simulink model "priority_01_prove"  (R2014b)
settings: Solver=FixedStepDiscrete  StartTime=0.0  StopTime=10.0  FixedStep=0.01  RelTol=1e-3
undefined symbols (not defined in the file): sldvsubsys
libraries: sldvlib x20, simulink x4
settings Model: Creator=Natasha  LastModifiedBy=JYOGANAN
settings DebuggingCC: UnderspecifiedInitializationDetection=Classic  MergeDetectMultiDrivingBlocksExec=none

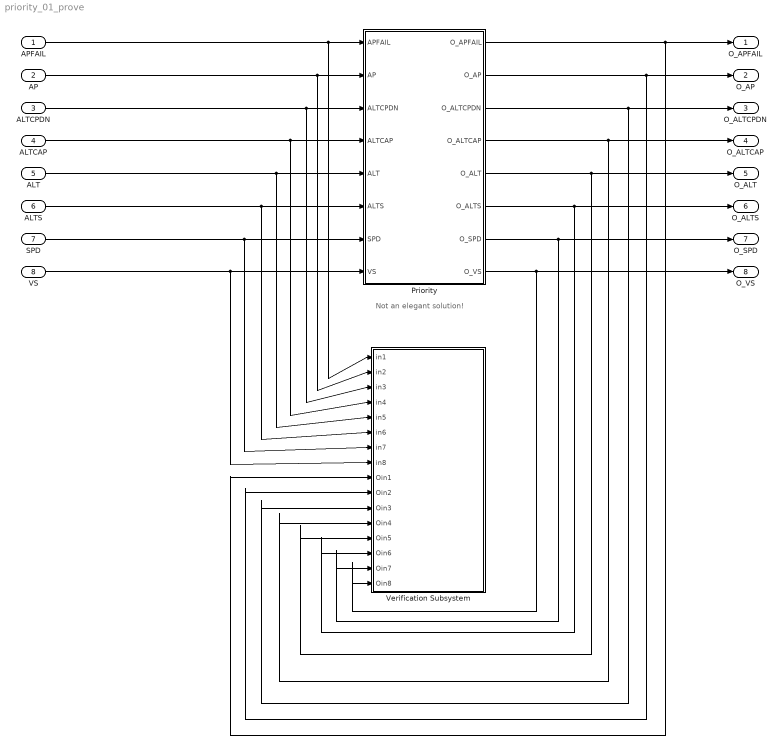
== system priority_01_prove ==
  note: Not an elegant
      | solution!
  APFAIL : Inport
  AP : Inport  Port=2
  ALTCPDN : Inport  Port=3
  ALTCAP : Inport  Port=4
  ALT : Inport  Port=5
  ALTS : Inport  Port=6
  SPD : Inport  Port=7
  VS : Inport  Port=8
  Priority : Subsystem
  Verification Subsystem : Subsystem  Tag=VerificationSubsystem  DisableCoverage=on  LoadFcn=sldvsubsys('check')  TreatAsAtomicUnit=on  SimViewingDevice=on  mask(VerificationSubsystem){}
      mask init:
      | sldvsubsys('maskInit');
      settings: CopyFcn=sldvsubsys('copy');  OpenFcn=open_system(gcb,'force');
      settings: PreSaveFcn=|
      | set_param(gcb,'SimViewingDevice','on');
      | sldvsubsys('check');
      mask Help: helpview(fullfile(docroot,'toolbox','sldv','sldv.map'),'verificationsubsystem')
      mask Display: image(imread('sldvicon_versubsys.png','BackGroundColor',[1 1 1]),'center');
  O_APFAIL : Outport
  O_AP : Outport  Port=2
  O_ALTCPDN : Outport  Port=3
  O_ALTCAP : Outport  Port=4
  O_ALT : Outport  Port=5
  O_ALTS : Outport  Port=6
  O_SPD : Outport  Port=7
  O_VS : Outport  Port=8
  wires:
  Priority/2(O_AP) -> Verification Subsystem/10(Oin2), O_AP/1
  Priority/3(O_ALTCPDN) -> Verification Subsystem/11(Oin3), O_ALTCPDN/1
  Priority/5(O_ALT) -> Verification Subsystem/13(Oin5), O_ALT/1
  Priority/1(O_APFAIL) -> Verification Subsystem/9(Oin1), O_APFAIL/1
  Priority/4(O_ALTCAP) -> Verification Subsystem/12(Oin4), O_ALTCAP/1
  Priority/6(O_ALTS) -> Verification Subsystem/14(Oin6), O_ALTS/1
  Priority/8(O_VS) -> Verification Subsystem/16(Oin8), O_VS/1
  ALT/1 -> Verification Subsystem/5(in5), Priority/5(ALT)
  APFAIL/1 -> Verification Subsystem/1(in1), Priority/1(APFAIL)
  AP/1 -> Verification Subsystem/2(in2), Priority/2(AP)
  ALTCAP/1 -> Verification Subsystem/4(in4), Priority/4(ALTCAP)
  ALTS/1 -> Verification Subsystem/6(in6), Priority/6(ALTS)
  SPD/1 -> Verification Subsystem/7(in7), Priority/7(SPD)
  VS/1 -> Verification Subsystem/8(in8), Priority/8(VS)
  ALTCPDN/1 -> Verification Subsystem/3(in3), Priority/3(ALTCPDN)
  Priority/7(O_SPD) -> Verification Subsystem/15(Oin7), O_SPD/1

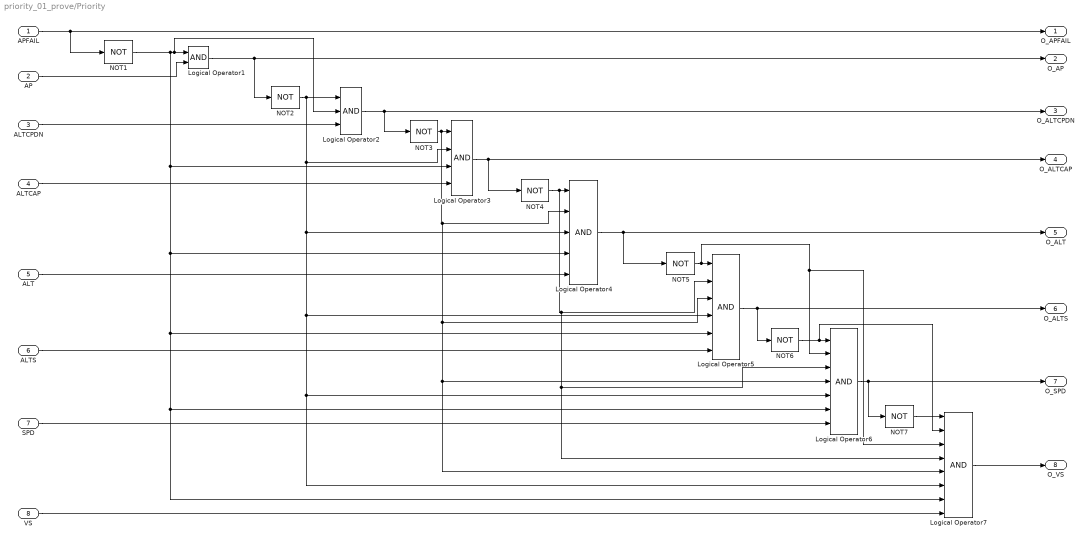
== system priority_01_prove/Priority ==
  APFAIL : Inport
  AP : Inport  Port=2
  ALTCPDN : Inport  Port=3
  ALTCAP : Inport  Port=4
  ALT : Inport  Port=5
  ALTS : Inport  Port=6
  SPD : Inport  Port=7
  VS : Inport  Port=8
  Logical Operator1 : Logic  AllPortsSameDT=off  OutDataTypeStr=boolean
  Logical Operator2 : Logic  Inputs=3  AllPortsSameDT=off  OutDataTypeStr=boolean
  Logical Operator3 : Logic  Inputs=4  AllPortsSameDT=off  OutDataTypeStr=boolean
  Logical Operator4 : Logic  Inputs=5  AllPortsSameDT=off  OutDataTypeStr=boolean
  Logical Operator5 : Logic  Inputs=6  AllPortsSameDT=off  OutDataTypeStr=boolean
  Logical Operator6 : Logic  Inputs=7  AllPortsSameDT=off  OutDataTypeStr=boolean
  Logical Operator7 : Logic  Inputs=8  AllPortsSameDT=off  OutDataTypeStr=boolean
  NOT{1..7} (7 alike) : Logic  Operator=NOT  AllPortsSameDT=off  OutDataTypeStr=boolean
  O_APFAIL : Outport
  O_AP : Outport  Port=2
  O_ALTCPDN : Outport  Port=3
  O_ALTCAP : Outport  Port=4
  O_ALT : Outport  Port=5
  O_ALTS : Outport  Port=6
  O_SPD : Outport  Port=7
  O_VS : Outport  Port=8
  wires:
  AP/1 -> Logical Operator1/2
  APFAIL/1 -> O_APFAIL/1, NOT1/1
  NOT1/1 -> Logical Operator2/2, Logical Operator1/1, Logical Operator3/3, Logical Operator4/4, Logical Operator5/5, Logical Operator6/6, Logical Operator7/7
  Logical Operator1/1 -> NOT2/1, O_AP/1
  ALTCPDN/1 -> Logical Operator2/3
  NOT2/1 -> Logical Operator7/6, Logical Operator6/5, Logical Operator5/4, Logical Operator4/3, Logical Operator3/2, Logical Operator2/1
  Logical Operator2/1 -> NOT3/1, O_ALTCPDN/1
  ALTCAP/1 -> Logical Operator3/4
  NOT3/1 -> Logical Operator7/5, Logical Operator6/4, Logical Operator5/3, Logical Operator4/2, Logical Operator3/1
  Logical Operator3/1 -> NOT4/1, O_ALTCAP/1
  NOT4/1 -> Logical Operator7/4, Logical Operator6/3, Logical Operator5/2, Logical Operator4/1
  ALT/1 -> Logical Operator4/5
  Logical Operator4/1 -> NOT5/1, O_ALT/1
  NOT5/1 -> Logical Operator7/3, Logical Operator6/2, Logical Operator5/1
  ALTS/1 -> Logical Operator5/6
  Logical Operator5/1 -> NOT6/1, O_ALTS/1
  NOT6/1 -> Logical Operator7/2, Logical Operator6/1
  SPD/1 -> Logical Operator6/7
  NOT7/1 -> Logical Operator7/1
  Logical Operator6/1 -> NOT7/1, O_SPD/1
  VS/1 -> Logical Operator7/8
  Logical Operator7/1 -> O_VS/1

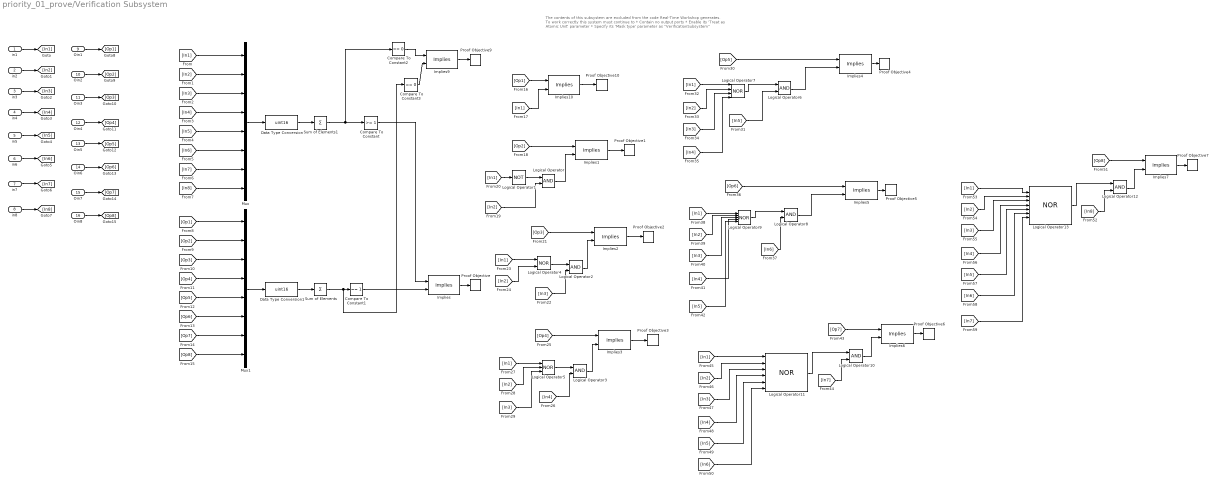
== system priority_01_prove/Verification Subsystem ==
  note: The contents of this subsystem are excluded from the code Real-Time
      | Workshop generates.
      |
      | To work correctly this system must continue to
      | * Contain no output ports
      | * Enable its 'Treat as Atomic Unit' parameter
      | * Specify its 'Mask type' parameter as "VerificationSubsystem"
  in1 : Inport
  in2 : Inport  Port=2
  in3 : Inport  Port=3
  in4 : Inport  Port=4
  in5 : Inport  Port=5
  in6 : Inport  Port=6
  in7 : Inport  Port=7
  in8 : Inport  Port=8
  Oin1 : Inport  Port=9
  Oin2 : Inport  Port=10
  Oin3 : Inport  Port=11
  Oin4 : Inport  Port=12
  Oin5 : Inport  Port=13
  Oin6 : Inport  Port=14
  Oin7 : Inport  Port=15
  Oin8 : Inport  Port=16
  Compare To Constant : simulink/Logic and Bit Operations/Compare To Constant  relop=>=  const=1  OutDataTypeStr=boolean
  Compare To Constant1 : simulink/Logic and Bit Operations/Compare To Constant  relop===  const=1  OutDataTypeStr=boolean
  Compare To Constant2 : simulink/Logic and Bit Operations/Compare To Constant  relop===  const=0  OutDataTypeStr=boolean
  Compare To Constant3 : simulink/Logic and Bit Operations/Compare To Constant  relop===  const=0  OutDataTypeStr=boolean
  Data Type Conversion : DataTypeConversion  OutDataTypeStr=uint16
  Data Type Conversion1 : DataTypeConversion  OutDataTypeStr=uint16
  Implies{,1..7,9..10} (10 alike) : sldvlib/Verification Utilities/Implies
  Logical Operator{,2..3,6,8,10,12} (7 alike) : Logic  AllPortsSameDT=off  OutDataTypeStr=boolean
  Logical Operator1 : Logic  Operator=NOT  AllPortsSameDT=off  OutDataTypeStr=boolean
  Logical Operator11 : Logic  Operator=NOR  Inputs=6  AllPortsSameDT=off  OutDataTypeStr=boolean
  Logical Operator13 : Logic  Operator=NOR  Inputs=7  AllPortsSameDT=off  OutDataTypeStr=boolean
  Logical Operator4 : Logic  Operator=NOR  AllPortsSameDT=off  OutDataTypeStr=boolean
  Logical Operator5 : Logic  Operator=NOR  Inputs=3  AllPortsSameDT=off  OutDataTypeStr=boolean
  Logical Operator7 : Logic  Operator=NOR  Inputs=4  AllPortsSameDT=off  OutDataTypeStr=boolean
  Logical Operator9 : Logic  Operator=NOR  Inputs=5  AllPortsSameDT=off  OutDataTypeStr=boolean
  Mux : Mux  Inputs=8
  Mux1 : Mux  Inputs=8
  Proof Objective{,1..7,9..10} (10 alike) : sldvlib/Objectives and Constraints/Proof Objective  enabled=on  customAVTBlockType=Proof Objective  intervals=true  dispValues=on  outEnabled=off  enableStopSim=off
      settings: AttributesFormatString=%<intervals>
  Sum of Elements : Sum  Inputs=+
  Sum of Elements1 : Sum  Inputs=+
  wires:
  Mux/1 -> Data Type Conversion/1
  Mux1/1 -> Data Type Conversion1/1
  Data Type Conversion1/1 -> Sum of Elements/1
  Data Type Conversion/1 -> Sum of Elements1/1
  Sum of Elements1/1 -> Compare To Constant2/1, Compare To Constant/1
  Sum of Elements/1 -> Compare To Constant3/1, Compare To Constant1/1
  Compare To Constant1/1 -> Implies/2
  Compare To Constant/1 -> Implies/1
  Implies/1 -> Proof Objective/1
  Implies9/1 -> Proof Objective9/1
  Compare To Constant2/1 -> Implies9/1
  Compare To Constant3/1 -> Implies9/2
  Implies10/1 -> Proof Objective10/1
  in1/1 -> [In1]
  in2/1 -> [In2]
  in3/1 -> [In3]
  in4/1 -> [In4]
  in5/1 -> [In5]
  in6/1 -> [In6]
  in7/1 -> [In7]
  in8/1 -> [In8]
  Oin1/1 -> [Op1]
  Oin2/1 -> [Op2]
  Oin3/1 -> [Op3]
  Oin4/1 -> [Op4]
  Oin5/1 -> [Op5]
  Oin6/1 -> [Op6]
  Oin7/1 -> [Op7]
  Oin8/1 -> [Op8]
  [In6] -> Mux/6
  [In5] -> Mux/5
  [In4] -> Mux/4
  [In8] -> Mux/8
  [In7] -> Mux/7
  [In3] -> Mux/3
  [In2] -> Mux/2
  [In1] -> Mux/1
  [Op6] -> Mux1/6
  [Op5] -> Mux1/5
  [Op4] -> Mux1/4
  [Op8] -> Mux1/8
  [Op7] -> Mux1/7
  [Op3] -> Mux1/3
  [Op2] -> Mux1/2
  [Op1] -> Mux1/1
  [Op1] -> Implies10/1
  [In1] -> Implies10/2
  Implies1/1 -> Proof Objective1/1
  [Op2] -> Implies1/1
  [In1] -> Logical Operator1/1
  [In2] -> Logical Operator/2
  Logical Operator/1 -> Implies1/2
  Logical Operator1/1 -> Logical Operator/1
  Implies2/1 -> Proof Objective2/1
  [Op3] -> Implies2/1
  [In3] -> Logical Operator2/2
  Logical Operator2/1 -> Implies2/2
  Logical Operator4/1 -> Logical Operator2/1
  [In1] -> Logical Operator4/1
  [In2] -> Logical Operator4/2
  Implies3/1 -> Proof Objective3/1
  [Op4] -> Implies3/1
  [In4] -> Logical Operator3/2
  Logical Operator3/1 -> Implies3/2
  Logical Operator5/1 -> Logical Operator3/1
  [In1] -> Logical Operator5/1
  [In2] -> Logical Operator5/2
  [In3] -> Logical Operator5/3
  Implies4/1 -> Proof Objective4/1
  [Op5] -> Implies4/1
  [In5] -> Logical Operator6/2
  Logical Operator6/1 -> Implies4/2
  Logical Operator7/1 -> Logical Operator6/1
  [In1] -> Logical Operator7/1
  [In2] -> Logical Operator7/2
  [In3] -> Logical Operator7/3
  [In4] -> Logical Operator7/4
  Implies5/1 -> Proof Objective5/1
  [Op6] -> Implies5/1
  [In6] -> Logical Operator8/2
  Logical Operator8/1 -> Implies5/2
  Logical Operator9/1 -> Logical Operator8/1
  [In1] -> Logical Operator9/1
  [In2] -> Logical Operator9/2
  [In3] -> Logical Operator9/3
  [In4] -> Logical Operator9/4
  [In5] -> Logical Operator9/5
  Implies6/1 -> Proof Objective6/1
  [Op7] -> Implies6/1
  [In7] -> Logical Operator10/2
  Logical Operator10/1 -> Implies6/2
  Logical Operator11/1 -> Logical Operator10/1
  [In1] -> Logical Operator11/1
  [In2] -> Logical Operator11/2
  [In3] -> Logical Operator11/3
  [In4] -> Logical Operator11/4
  [In5] -> Logical Operator11/5
  [In6] -> Logical Operator11/6
  Implies7/1 -> Proof Objective7/1
  [Op8] -> Implies7/1
  [In8] -> Logical Operator12/2
  Logical Operator12/1 -> Implies7/2
  Logical Operator13/1 -> Logical Operator12/1
  [In1] -> Logical Operator13/1
  [In2] -> Logical Operator13/2
  [In3] -> Logical Operator13/3
  [In4] -> Logical Operator13/4
  [In5] -> Logical Operator13/5
  [In6] -> Logical Operator13/6
  [In7] -> Logical Operator13/7
